simulink model "Buck_converter_dcdc"  (R2025a)
settings: Solver=ode23t  StartTime=0.0  StopTime=.10  MaxStep=1e-6  RelTol=1e-3
libraries: spsSeriesRLCBranchLib x4, spsVoltageMeasurementLib x2, spsDCVoltageSourceLib x1, spsDiodeLib x1, spsIdealSwitchLib x1, spsMosfetLib x1, simulink x1, spsCurrentMeasurementLib x1, sps_lib x1

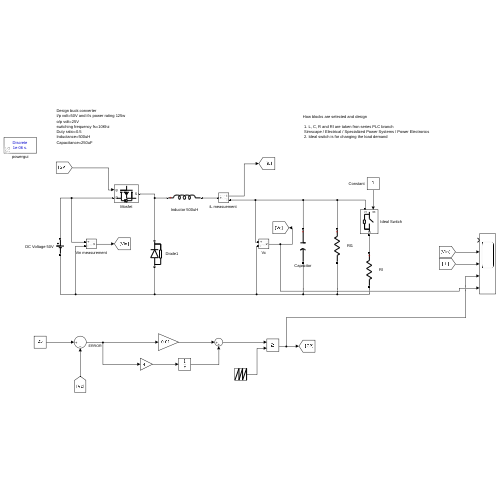
[thumbnail: Simulink's stored preview of the top-level diagram]
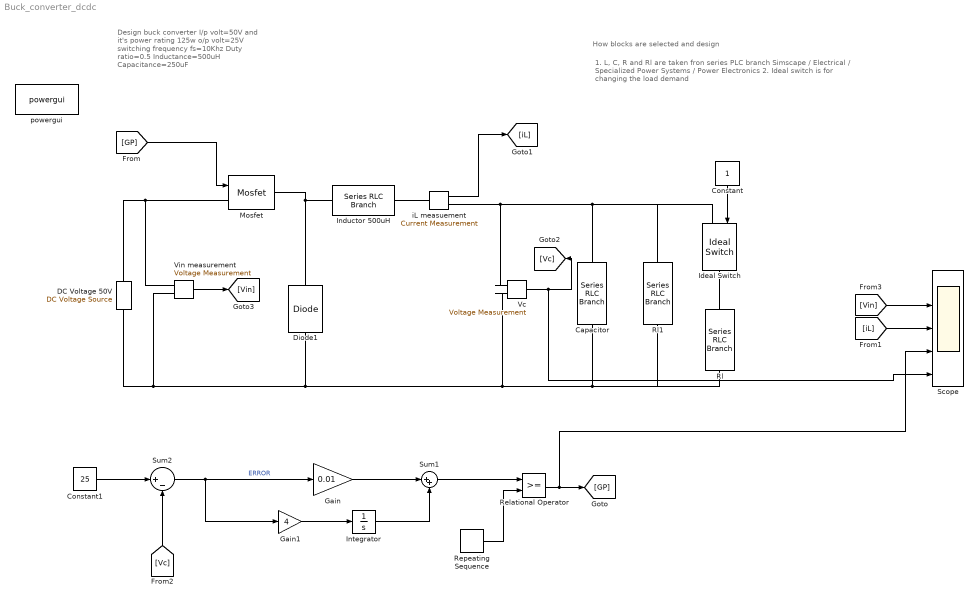
== system Buck_converter_dcdc ==
  note: 1. L, C, R and Rl are taken fron series PLC branch
      | Simscape / Electrical / Specialized Power Systems / Power Electronics
      | 2. Ideal switch is for changing the load demand
  note: How blocks are selected and design
  note: Design buck converter
      | I/p volt=50V and it's power rating 125w
      | o/p volt=25V
      | switching frequency fs=10Khz
      | Duty ratio=0.5
      | Inductance=500uH
      | Capacitance=250uF
  Capacitor : spsSeriesRLCBranchLib/Series RLC Branch  LConnTagsString=__new0  RConnTagsString=__new0  BranchType=C  Resistance=1  Inductance=1e-3  SetiL0=off  InitialCurrent=0  Capacitance=250e-6  Setx0=off  InitialVoltage=0  Measurements=None
  Constant : Constant
  Constant1 : Constant  Value=25
  DC Voltage 50V : spsDCVoltageSourceLib/DC Voltage Source  Amplitude=50  Measurements=None
  Diode1 : spsDiodeLib/Diode  Ron=0.001  Lon=0  Vf=0.8  IC=0  UseSnubber=off  Rs=50000  Cs=250e-9  Measurements=off
  Gain : Gain  Gain=0.01
  Gain1 : Gain  Gain=4
  Ideal Switch : spsIdealSwitchLib/Ideal Switch  Ron=0.001  Lon=0  IC=0  Rs=1e5  Cs=inf  Measurements=off
  Inductor 500uH : spsSeriesRLCBranchLib/Series RLC Branch  LConnTagsString=__new0  RConnTagsString=__new0  BranchType=L  Resistance=1  Inductance=500e-6  SetiL0=off  InitialCurrent=0  Capacitance=1e-6  Setx0=off  InitialVoltage=0  Measurements=None
  Integrator : Integrator
  Mosfet : spsMosfetLib/Mosfet  Ron=0.1  Lon=0  Rd=0.01  Vfd=0  IC=0  Rs=1e5  Cs=inf  Measurements=off
  Relational Operator : RelationalOperator  OutDataTypeStr=boolean  RndMeth=Simplest  InputSameDT=off
  Repeating Sequence : simulink/Sources/Repeating Sequence  rep_seq_t=[0 1]/10000  rep_seq_y=[0 2]
  Rl : spsSeriesRLCBranchLib/Series RLC Branch  LConnTagsString=__new0  RConnTagsString=__new0  BranchType=R  Resistance=1  Inductance=1e-3  SetiL0=off  InitialCurrent=0  Capacitance=1e-6  Setx0=off  InitialVoltage=0  Measurements=None
  Rl1 : spsSeriesRLCBranchLib/Series RLC Branch  LConnTagsString=__new0  RConnTagsString=__new0  BranchType=R  Resistance=5  Inductance=1e-3  SetiL0=off  InitialCurrent=0  Capacitance=1e-6  Setx0=off  InitialVoltage=0  Measurements=None
  Scope : Scope  NumInputPorts=5
      settings: ActiveDisplayYMinimum=-40.788919223803362  ActiveDisplayYMaximum=53.550295019746926
  Sum1 : Sum  Inputs=|++
  Sum2 : Sum  Inputs=|+-
  Vc : spsVoltageMeasurementLib/Voltage Measurement  PhasorSimulation=off  OutputType=Complex  PSBequivalent=0
  Vin measurement : spsVoltageMeasurementLib/Voltage Measurement  PhasorSimulation=off  OutputType=Complex  PSBequivalent=0
  "iL measuement " : spsCurrentMeasurementLib/Current Measurement  PhasorSimulation=off  OutputType=Complex  PSBequivalent=0
  powergui : sps_lib/powergui  Priority=1  SimulationMode=Discrete  SampleTime=1e-06  frequency=60  Iterations=50  frequencyindice=0  Pbase=100e6  ErrMax=1e-4  UnitsV=kV  UnitsW=MW  buscounter=0  FunctionMessages=off  echomessages=off  EnableUseOfTLC=off  CurrentSourceSwitches=off  DisableSnubberDevices=off  DisableRonSwitches=off  DisableVfSwitches=off  DisplayEquations=off  AutomaticDiscreteSolvers=off  SolverType=Tustin/Backward Euler (TBE)  Interpol=off  ExternalGateDelay=off  methode=off  Ts=100  x0status=blocks  SPID=on  SwTol=0  HookPort=off  NonlinearTolerance=1e-4  nMaxIteration=100  ContinueOnMaxIteration=off  RestoreLinks=warning  ResistiveCurrentMeasurement=off  Frange=[0:2:500]  Ylog=off  Xlog=on  ShowGrid=off  save=off  variable=ZData  structure=0  ZoomFFT=off  StartTime=0.0  cycles=1  DisplayStyle=1  fundamental=60  FreqAxis=off  MaxFrequency=1000  frequencyindicesteady=1  RmsSteady=1  display=off
  wires:
  [GP] -> Mosfet/1
  "iL measuement "/1 -> [iL]
  Vc/1 -> Scope/5, [Vc]
  Constant/1 -> Ideal Switch/1
  Vin measurement/1 -> [Vin]
  [Vc] -> Sum2/2
  Gain1/1 -> Integrator/1
  Sum2/1 -> Gain1/1, Gain/1  "ERROR"
  Gain/1 -> Sum1/1
  Integrator/1 -> Sum1/2
  Sum1/1 -> Relational Operator/1
  Repeating Sequence/1 -> Relational Operator/2
  Relational Operator/1 -> Scope/4, [GP]
  Constant1/1 -> Sum2/1
  [Vin] -> Scope/2
  [iL] -> Scope/3
  connections:
  DC Voltage 50V/RConn1 -- Vin measurement/LConn1 -- Mosfet/LConn1
  Inductor 500uH/LConn1 -- Diode1/RConn1 -- Mosfet/RConn1
  "iL measuement "/LConn1 -- Inductor 500uH/RConn1
  "iL measuement "/RConn1 -- Vc/LConn1 -- Rl1/LConn1 -- Ideal Switch/LConn1 -- Capacitor/LConn1
  DC Voltage 50V/LConn1 -- Vin measurement/LConn2 -- Diode1/LConn1 -- Vc/LConn2 -- Rl1/RConn1 -- Rl/RConn1 -- Capacitor/RConn1
  Ideal Switch/RConn1 -- Rl/LConn1
